simulink model "ES241A_MotAg2Meas"
settings: Solver=FixedStepDiscrete  SolverMode=SingleTasking  StartTime=0.0  StopTime=1  FixedStep=0.002  RelTol=1e-3
values from neighbouring files (symbols this model uses):
  ARCHGLBPRM_2PI_ULS_F32 = DataDict.Constant    [ES241A_MotAg2Meas_DataDict.m]
  FLTINJ_MOTAG2MEAS_MOTAG2MECL = DataDict.Constant    [ES241A_MotAg2Meas_DataDict.m]
  MOTAG2ANSINCOSFLTFAILSTEP_CNT_U16 = DataDict.Constant    [ES241A_MotAg2Meas_DataDict.m]
  MOTAG2ANSINCOSFLTPASSSTEP_CNT_U16 = DataDict.Constant    [ES241A_MotAg2Meas_DataDict.m]
  MotAg2MeasOffs = DataDict.Calibration    [ES241A_MotAg2Meas_DataDict.m]
  MOTAG2MECLMAX_MOTREV_F32 = DataDict.Constant    [ES241A_MotAg2Meas_DataDict.m]
  MOTAG2MECLMIN_MOTREV_F32 = DataDict.Constant    [ES241A_MotAg2Meas_DataDict.m]
  VALMAXERR_VOLTSQD_F32 = DataDict.Constant    [ES241A_MotAg2Meas_DataDict.m]
  VALMINERR_VOLTSQD_F32 = DataDict.Constant    [ES241A_MotAg2Meas_DataDict.m]
undefined symbols (not defined in the file or in its folder): NtcNr1, NtcSts1, sigbuilder_block
libraries: simulink x12, NxtrLim x2, FloatToFixd x1, NxtrMath x1
(part 2 of 3)

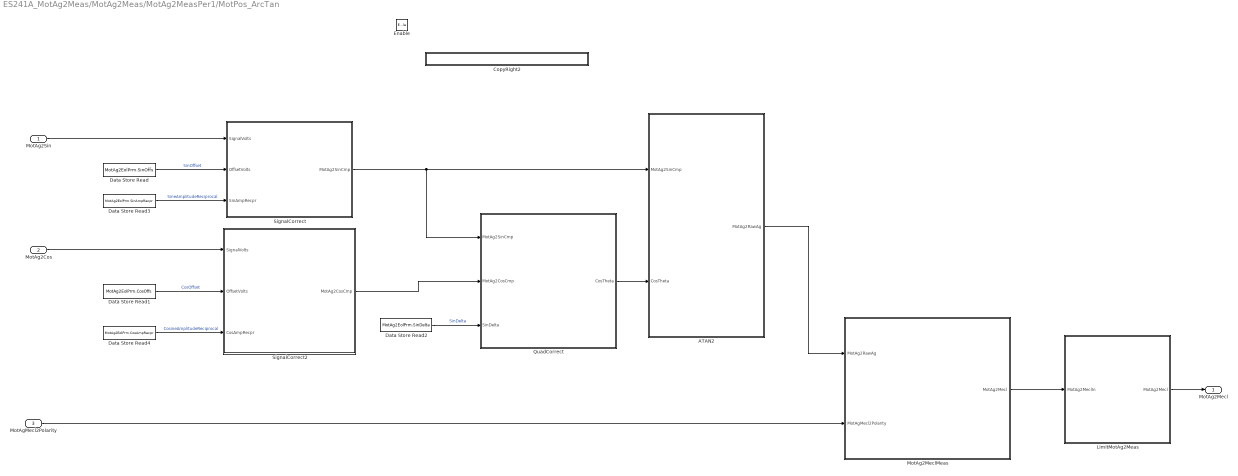
== system ES241A_MotAg2Meas/MotAg2Meas/MotAg2MeasPer1/MotPos_ArcTan ==
  MotAg2Sin : Inport
  MotAg2Cos : Inport  Port=2
  MotAgMecl2Polarity : Inport  RequirementInfo={} %GIDa_f88c60fe_1722_4e27_ab61_8a7da6a73543  Port=3
  Enable : EnablePort
  ATAN2 : Subsystem  RequirementInfo={'linktype_rmi_doors' '0000cf65 (/E-STEER Core/SubSystem Specifications/Electrical Actuator/Control Module/FDD Module Requirements/EA4/ES241A_MotAg2Meas)' '#ES241A_123' 'true' 'REQ: ES241A_123' '' } %GIDa_4a37e0cf_c570_47cf_a8a6_a1060e3c63ea  TreatAsAtomicUnit=on
  CopyRight2 : Subsystem  Description=|  mask(Copyright Information){none=on}
      | Copyright info block.                                               
      |                                                                     
      | Place copyright information at the top of every subsystem in design.
      mask prompts: none "No parameters"
      mask help: Place copyright information at the top of every subsystem in design.
      mask Display:
      | NxtrConf = 'Nexteer Confidential';
      | 
      | sys = bdroot; %handle for the current model ("system")
      | first = get_param(sys,'Created');
      | if(isempty(first))
      |     first = datestr(now,'yyyy');
      | else
      |     first = first(end-3:end);  %year is last four digits
      | end
      | 
      | last = get_param(sys,'LastModifiedDate');
      | if isempty(last)
      |     last = datestr(now,'yyyy');
      | else
      |     last = last(end-3:end);
      | end
      | 
      | if strcmp(first,last)
      |     fprintf('%s -- Copyright %s Nexteer',NxtrConf,first)
      | else
      |     fprintf('%s -- %s%s- %s Nexteer',NxtrConf,char(169),first,last)
      | end
  Data Store Read : DataStoreRead  DataStoreName=MotAg2EolPrm  DataStoreElements=MotAg2EolPrm.SinOffs
  Data Store Read1 : DataStoreRead  DataStoreName=MotAg2EolPrm  DataStoreElements=MotAg2EolPrm.CosOffs
  Data Store Read2 : DataStoreRead  DataStoreName=MotAg2EolPrm  DataStoreElements=MotAg2EolPrm.SinDelta
  Data Store Read3 : DataStoreRead  DataStoreName=MotAg2EolPrm  DataStoreElements=MotAg2EolPrm.SinAmpRecpr
  Data Store Read4 : DataStoreRead  DataStoreName=MotAg2EolPrm  DataStoreElements=MotAg2EolPrm.CosAmpRecpr
  LimitMotAg2Meas : Subsystem
  MotAg2MeclMeas : Subsystem  RequirementInfo="{}  %GIDa_155eb0a8_c2ed_490a_af1d_f8f4e19f97e7"  TreatAsAtomicUnit=on
  QuadCorrect : Subsystem  RequirementInfo={'linktype_rmi_doors' '0000cf65 (/E-STEER Core/SubSystem Specifications/Electrical Actuator/Control Module/FDD Module Requirements/EA4/ES241A_MotAg2Meas)' '#ES241A_121' 'true' 'REQ: ES241A_121' '' } %GIDa_3d78f2b2_5c94_409f_934c_8aefaaebd76d  TreatAsAtomicUnit=on
  SignalCorrect : Subsystem  RequirementInfo={'linktype_rmi_doors' '0000cf65 (/E-STEER Core/SubSystem Specifications/Electrical Actuator/Control Module/FDD Module Requirements/EA4/ES241A_MotAg2Meas)' '#ES241A_117' 'true' 'REQ: ES241A_117' '' } %GIDa_8d0c5619_ebe6_40e3_89d6_85a8ef0fbaf9
  SignalCorrect2 : Subsystem  RequirementInfo={'linktype_rmi_doors' '0000cf65 (/E-STEER Core/SubSystem Specifications/Electrical Actuator/Control Module/FDD Module Requirements/EA4/ES241A_MotAg2Meas)' '#ES241A_83' 'true' 'REQ: ES241A_83' '' } %GIDa_07f3fc20_adc4_4d19_a2a9_4772ed53a785
  MotAg2Mecl : Outport  RequirementInfo="{}  %GIDa_dd9bd2af_a5c1_4575_89a6_d173bd83c2f9"
  wires:
  SignalCorrect/1(MotAg2SinCmp) -> QuadCorrect/1(MotAg2SinCmp), ATAN2/1(MotAg2SinCmp)
  ATAN2/1(MotAg2RawAg) -> MotAg2MeclMeas/1(MotAg2RawAg)
  MotAg2Cos/1 -> SignalCorrect2/1(SignalVolts)
  MotAgMecl2Polarity/1 -> MotAg2MeclMeas/2(MotAgMecl2Polarity)
  SignalCorrect2/1(MotAg2CosCmp) -> QuadCorrect/2(MotAg2CosCmp)
  Data Store Read/1 -> SignalCorrect/2(OffsetVolts)  "SinOffset"
  Data Store Read3/1 -> SignalCorrect/3(SinAmpRecpr)  "SineAmplitudeReciprocal"
  Data Store Read1/1 -> SignalCorrect2/2(OffsetVolts)  "CosOffset"
  Data Store Read4/1 -> SignalCorrect2/3(CosAmpRecpr)  "CosineAmplitudeReciprocal"
  Data Store Read2/1 -> QuadCorrect/3(SinDelta)  "SinDelta"
  MotAg2Sin/1 -> SignalCorrect/1(SignalVolts)
  MotAg2MeclMeas/1(MotAg2Mecl) -> LimitMotAg2Meas/1(MotAg2MeclIn)
  LimitMotAg2Meas/1(MotAg2Mecl) -> MotAg2Mecl/1
  QuadCorrect/1(CosTheta) -> ATAN2/2(CosTheta)

== system ES241A_MotAg2Meas/MotAg2Meas/MotAg2MeasInit1/MotAg2EolPrm_GetErrorStatus/CopyRight2 ==

== system ES241A_MotAg2Meas/MotAg2Meas/MotAg2MeasInit1/NVM_NOK/CopyRight2 ==

== system ES241A_MotAg2Meas/MotAg2Meas/MotAg2MeasInit1/NVM_Ok/CopyRight2 ==

== system ES241A_MotAg2Meas/MotAg2Meas/MotAg2MeasPer1/AnalogMsbDiagnostics/CopyRight2 ==

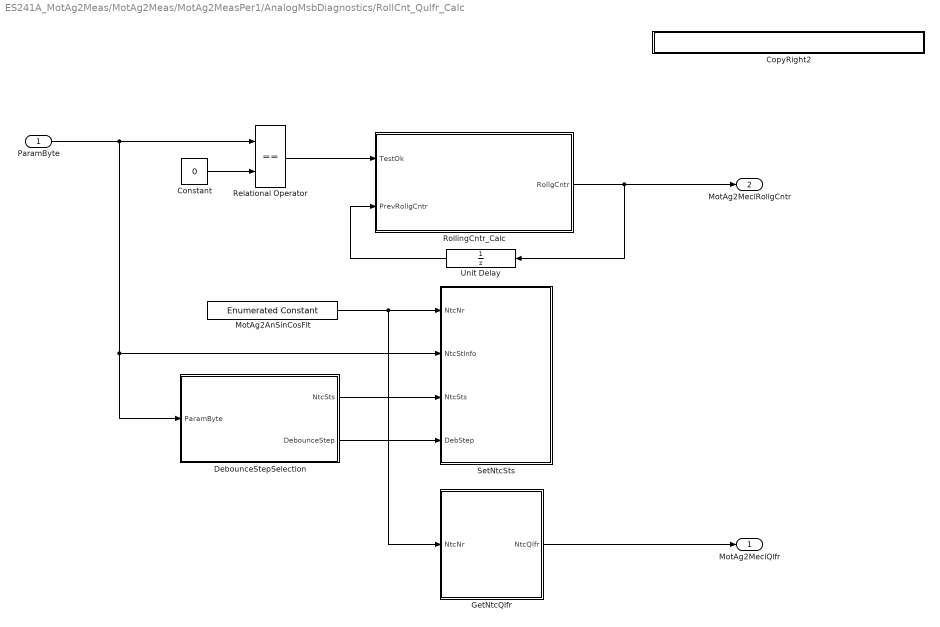
== system ES241A_MotAg2Meas/MotAg2Meas/MotAg2MeasPer1/AnalogMsbDiagnostics/RollCnt_Qulfr_Calc ==
  ParamByte : Inport
  Constant : Constant  Value=0
  CopyRight2 : Subsystem  Description=|  mask(Copyright Information){none=on}
      | Copyright info block.                                               
      |                                                                     
      | Place copyright information at the top of every subsystem in design.
      mask prompts: none "No parameters"
      mask help: Place copyright information at the top of every subsystem in design.
      mask Display:
      | NxtrConf = 'Nexteer Confidential';
      | 
      | sys = bdroot; %handle for the current model ("system")
      | first = get_param(sys,'Created');
      | if(isempty(first))
      |     first = datestr(now,'yyyy');
      | else
      |     first = first(end-3:end);  %year is last four digits
      | end
      | 
      | last = get_param(sys,'LastModifiedDate');
      | if isempty(last)
      |     last = datestr(now,'yyyy');
      | else
      |     last = last(end-3:end);
      | end
      | 
      | if strcmp(first,last)
      |     fprintf('%s -- Copyright %s Nexteer',NxtrConf,first)
      | else
      |     fprintf('%s -- %s%s- %s Nexteer',NxtrConf,char(169),first,last)
      | end
  DebounceStepSelection : Subsystem
  GetNtcQlfr : Subsystem  RequirementInfo={'linktype_rmi_doors' '0000cf65 (/E-STEER Core/SubSystem Specifications/Electrical Actuator/Control Module/FDD Module Requirements/EA4/ES241A_MotAg2Meas)' '#ES241A_136' 'true' 'REQ: ES241A_136' '' } %GIDa_6b67fe78_f19c_4eda_b14f_32aa673a2169
  MotAg2AnSinCosFlt : simulink/Sources/Enumerated Constant  OutDataTypeStr=Enum: NtcNr1  Value=NtcNr1.NTCNR_0X087  SampleTime=inf
  Relational Operator : RelationalOperator  Operator===  OutDataTypeStr=boolean
  RollingCntr_Calc : Stateflow chart  TreatAsAtomicUnit=on
  SetNtcSts : Subsystem  RequirementInfo={} %GIDa_9fe419b1_aead_4464_8eaa_fcc4c094b192
  Unit Delay : UnitDelay  SampleTime=-1  StateName=MotAg2MeclRollgCntrPrev  StateMustResolveToSignalObject=on
      settings: AttributesFormatString=%<StateName>
  MotAg2MeclQlfr : Outport
  MotAg2MeclRollgCntr : Outport  Port=2
  wires:
  ParamByte/1 -> Relational Operator/1, DebounceStepSelection/1(ParamByte), SetNtcSts/2(NtcStInfo)
  RollingCntr_Calc/1(RollgCntr) -> MotAg2MeclRollgCntr/1, Unit Delay/1
  DebounceStepSelection/2(DebounceStep) -> SetNtcSts/4(DebStep)
  MotAg2AnSinCosFlt/1 -> GetNtcQlfr/1(NtcNr), SetNtcSts/1(NtcNr)
  GetNtcQlfr/1(NtcQlfr) -> MotAg2MeclQlfr/1
  DebounceStepSelection/1(NtcSts) -> SetNtcSts/3(NtcSts)
  Relational Operator/1 -> RollingCntr_Calc/1(TestOk)
  Constant/1 -> Relational Operator/2
  Unit Delay/1 -> RollingCntr_Calc/2(PrevRollgCntr)

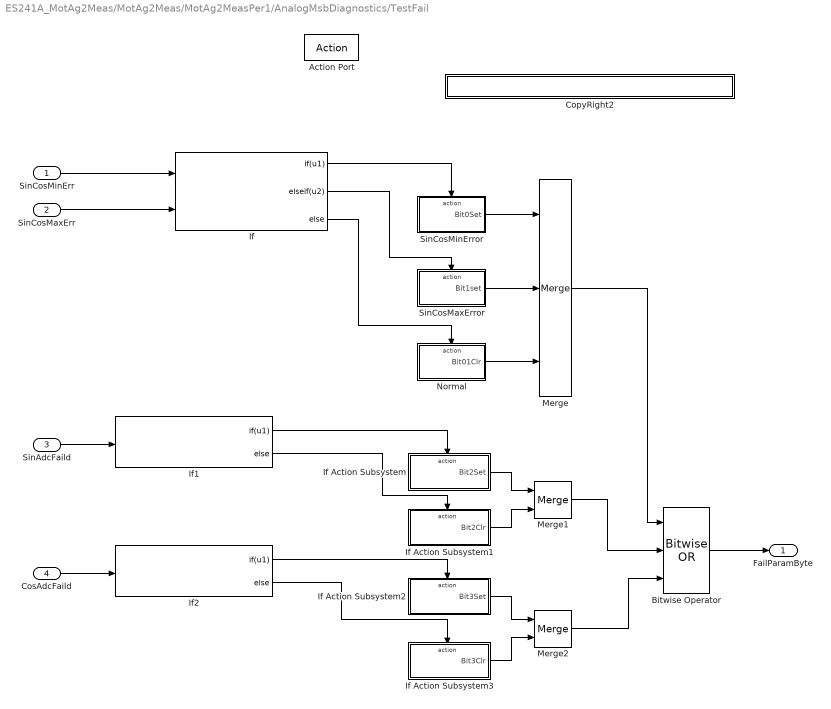
== system ES241A_MotAg2Meas/MotAg2Meas/MotAg2MeasPer1/AnalogMsbDiagnostics/TestFail ==
  SinCosMinErr : Inport
  SinCosMaxErr : Inport  Port=2
  SinAdcFaild : Inport  Port=3
  CosAdcFaild : Inport  Port=4
  Action Port : ActionPort  ActionType=then
  Bitwise Operator : simulink/Logic and Bit Operations/Bitwise Operator  logicop=OR  UseBitMask=off  NumInputPorts=3  BitMask=bin2dec('11011001')  BitMaskRealWorld=Stored Integer
  CopyRight2 : Subsystem  Description=|  mask(Copyright Information){none=on}
      | Copyright info block.                                               
      |                                                                     
      | Place copyright information at the top of every subsystem in design.
      mask prompts: none "No parameters"
      mask help: Place copyright information at the top of every subsystem in design.
      mask Display:
      | NxtrConf = 'Nexteer Confidential';
      | 
      | sys = bdroot; %handle for the current model ("system")
      | first = get_param(sys,'Created');
      | if(isempty(first))
      |     first = datestr(now,'yyyy');
      | else
      |     first = first(end-3:end);  %year is last four digits
      | end
      | 
      | last = get_param(sys,'LastModifiedDate');
      | if isempty(last)
      |     last = datestr(now,'yyyy');
      | else
      |     last = last(end-3:end);
      | end
      | 
      | if strcmp(first,last)
      |     fprintf('%s -- Copyright %s Nexteer',NxtrConf,first)
      | else
      |     fprintf('%s -- %s%s- %s Nexteer',NxtrConf,char(169),first,last)
      | end
  If : If  RequirementInfo={} %GIDa_a9e4a426_b13f_48ac_85a4_f1708270da02  NumInputs=2  IfExpression=u1  ElseIfExpressions=u2
  If Action Subsystem : Subsystem  RequirementInfo={'linktype_rmi_doors' '0000cf65 (/E-STEER Core/SubSystem Specifications/Electrical Actuator/Control Module/FDD Module Requirements/EA4/ES241A_MotAg2Meas)' '#ES241A_149' 'true' 'REQ: ES241A_149' '' } %GIDa_afb555f9_4864_4292_98a1_720bafda0c91  TreatAsAtomicUnit=on
  If Action Subsystem1 : Subsystem  RequirementInfo={'linktype_rmi_doors' '0000cf65 (/E-STEER Core/SubSystem Specifications/Electrical Actuator/Control Module/FDD Module Requirements/EA4/ES241A_MotAg2Meas)' '#ES241A_149' 'true' 'REQ: ES241A_149' '' } %GIDa_7a5d096e_f46e_4b81_973a_a988b07ea5da  TreatAsAtomicUnit=on
  If Action Subsystem2 : Subsystem  RequirementInfo={'linktype_rmi_doors' '0000cf65 (/E-STEER Core/SubSystem Specifications/Electrical Actuator/Control Module/FDD Module Requirements/EA4/ES241A_MotAg2Meas)' '#ES241A_150' 'true' 'REQ: ES241A_150' '' } %GIDa_1a2e8224_376f_4f7e_a8de_e2f9f89e8409  TreatAsAtomicUnit=on
  If Action Subsystem3 : Subsystem  RequirementInfo={'linktype_rmi_doors' '0000cf65 (/E-STEER Core/SubSystem Specifications/Electrical Actuator/Control Module/FDD Module Requirements/EA4/ES241A_MotAg2Meas)' '#ES241A_150' 'true' 'REQ: ES241A_150' '' } %GIDa_804518a5_ac45_4ee5_ad42_fdad3805a040  TreatAsAtomicUnit=on
  If1 : If  RequirementInfo={} %GIDa_4ac208ba_4fea_48e5_9089_44454d5bb31e  IfExpression=u1
  If2 : If  RequirementInfo={} %GIDa_95f3580d_6d83_47db_9291_d4b911f8f78c  IfExpression=u1
  Merge : Merge  Inputs=3
  Merge1 : Merge
  Merge2 : Merge
  Normal : Subsystem  RequirementInfo={'linktype_rmi_doors' '0000cf65 (/E-STEER Core/SubSystem Specifications/Electrical Actuator/Control Module/FDD Module Requirements/EA4/ES241A_MotAg2Meas)' '#ES241A_132' 'true' 'REQ: ES241A_132' '' ; 'linktype_rmi_doors' '0000cf65 (/E-STEER Core/SubSystem Specifications/Electrical Actuator/Control Module/FDD Module Requirements/EA4/ES241A_MotAg2Meas)' '#ES241A_133' 'true' 'REQ: ES241A_133' '' } %GIDa_7888af4c_2405_41f3_8422_50cb1e840d88  TreatAsAtomicUnit=on
  SinCosMaxError : Subsystem  RequirementInfo={'linktype_rmi_doors' '0000cf65 (/E-STEER Core/SubSystem Specifications/Electrical Actuator/Control Module/FDD Module Requirements/EA4/ES241A_MotAg2Meas)' '#ES241A_132' 'true' 'REQ: ES241A_132' '' } %GIDa_2a13378d_a5ac_4539_9cf9_334d2a433c6e  TreatAsAtomicUnit=on
  SinCosMinError : Subsystem  RequirementInfo={'linktype_rmi_doors' '0000cf65 (/E-STEER Core/SubSystem Specifications/Electrical Actuator/Control Module/FDD Module Requirements/EA4/ES241A_MotAg2Meas)' '#ES241A_133' 'true' 'REQ: ES241A_133' '' } %GIDa_e3821827_fad7_4466_9101_6350f28db25f  TreatAsAtomicUnit=on
  FailParamByte : Outport
  wires:
  SinCosMinErr/1 -> If/1
  If/1 -> SinCosMinError/Action
  SinCosMinError/1(Bit0Set) -> Merge/1
  SinCosMaxError/1(Bit1set) -> Merge/2
  SinCosMaxErr/1 -> If/2
  If/2 -> SinCosMaxError/Action
  SinAdcFaild/1 -> If1/1
  CosAdcFaild/1 -> If2/1
  If/3 -> Normal/Action
  Normal/1(Bit01Clr) -> Merge/3
  If1/1 -> If Action Subsystem/Action
  If1/2 -> If Action Subsystem1/Action
  If2/1 -> If Action Subsystem2/Action
  If2/2 -> If Action Subsystem3/Action
  If Action Subsystem/1(Bit2Set) -> Merge1/1
  If Action Subsystem1/1(Bit2Clr) -> Merge1/2
  If Action Subsystem2/1(Bit3Set) -> Merge2/1
  If Action Subsystem3/1(Bit3Clr) -> Merge2/2
  Merge1/1 -> Bitwise Operator/2
  Merge2/1 -> Bitwise Operator/3
  Bitwise Operator/1 -> FailParamByte/1
  Merge/1 -> Bitwise Operator/1

== system ES241A_MotAg2Meas/MotAg2Meas/MotAg2MeasPer1/AnalogMsbDiagnostics/TestPass ==
  Action Port : ActionPort  ActionType=else
  Constant : Constant  Value=0  OutDataTypeStr=uint8
      settings: AttributesFormatString=%<OutDataTypeStr>
  CopyRight2 : Subsystem  Description=|  mask(Copyright Information){none=on}
      | Copyright info block.                                               
      |                                                                     
      | Place copyright information at the top of every subsystem in design.
      mask prompts: none "No parameters"
      mask help: Place copyright information at the top of every subsystem in design.
      mask Display:
      | NxtrConf = 'Nexteer Confidential';
      | 
      | sys = bdroot; %handle for the current model ("system")
      | first = get_param(sys,'Created');
      | if(isempty(first))
      |     first = datestr(now,'yyyy');
      | else
      |     first = first(end-3:end);  %year is last four digits
      | end
      | 
      | last = get_param(sys,'LastModifiedDate');
      | if isempty(last)
      |     last = datestr(now,'yyyy');
      | else
      |     last = last(end-3:end);
      | end
      | 
      | if strcmp(first,last)
      |     fprintf('%s -- Copyright %s Nexteer',NxtrConf,first)
      | else
      |     fprintf('%s -- %s%s- %s Nexteer',NxtrConf,char(169),first,last)
      | end
  PassParamByte : Outport
  wires:
  Constant/1 -> PassParamByte/1  "ParamByte"

== system ES241A_MotAg2Meas/MotAg2Meas/MotAg2MeasPer1/FltInj_f32/CopyRight2 ==

== system ES241A_MotAg2Meas/MotAg2Meas/MotAg2MeasPer1/MotAngleMechRevJdgmnt/CopyRight2 ==

== system ES241A_MotAg2Meas/MotAg2Meas/MotAg2MeasPer1/MotAngleMechRevJdgmnt/TesOk_Fail ==
  In1 : Inport
  Action Port : ActionPort  ActionType=else
  CopyRight2 : Subsystem  Description=|  mask(Copyright Information){none=on}
      | Copyright info block.                                               
      |                                                                     
      | Place copyright information at the top of every subsystem in design.
      mask prompts: none "No parameters"
      mask help: Place copyright information at the top of every subsystem in design.
      mask Display:
      | NxtrConf = 'Nexteer Confidential';
      | 
      | sys = bdroot; %handle for the current model ("system")
      | first = get_param(sys,'Created');
      | if(isempty(first))
      |     first = datestr(now,'yyyy');
      | else
      |     first = first(end-3:end);  %year is last four digits
      | end
      | 
      | last = get_param(sys,'LastModifiedDate');
      | if isempty(last)
      |     last = datestr(now,'yyyy');
      | else
      |     last = last(end-3:end);
      | end
      | 
      | if strcmp(first,last)
      |     fprintf('%s -- Copyright %s Nexteer',NxtrConf,first)
      | else
      |     fprintf('%s -- %s%s- %s Nexteer',NxtrConf,char(169),first,last)
      | end
  Out1 : Outport
  wires:
  In1/1 -> Out1/1

== system ES241A_MotAg2Meas/MotAg2Meas/MotAg2MeasPer1/MotAngleMechRevJdgmnt/TesOk_Pass ==
  In1 : Inport
  Action Port : ActionPort  ActionType=then
  CopyRight2 : Subsystem  Description=|  mask(Copyright Information){none=on}
      | Copyright info block.                                               
      |                                                                     
      | Place copyright information at the top of every subsystem in design.
      mask prompts: none "No parameters"
      mask help: Place copyright information at the top of every subsystem in design.
      mask Display:
      | NxtrConf = 'Nexteer Confidential';
      | 
      | sys = bdroot; %handle for the current model ("system")
      | first = get_param(sys,'Created');
      | if(isempty(first))
      |     first = datestr(now,'yyyy');
      | else
      |     first = first(end-3:end);  %year is last four digits
      | end
      | 
      | last = get_param(sys,'LastModifiedDate');
      | if isempty(last)
      |     last = datestr(now,'yyyy');
      | else
      |     last = last(end-3:end);
      | end
      | 
      | if strcmp(first,last)
      |     fprintf('%s -- Copyright %s Nexteer',NxtrConf,first)
      | else
      |     fprintf('%s -- %s%s- %s Nexteer',NxtrConf,char(169),first,last)
      | end
  Out1 : Outport
  wires:
  In1/1 -> Out1/1

== system ES241A_MotAg2Meas/MotAg2Meas/MotAg2MeasPer1/MotPos_ArcTan/ATAN2 ==
  note: The motor angle mechanical output is 0 to 1 motor mechancial revolutions.
      |  Zero represents the point where sine is 0 and cosine is 1
  MotAg2SinCmp : Inport
  CosTheta : Inport  Port=2
  Arctan2_f32 : NxtrMath/Arctan2_f32  SFunctionSpec=single y1 = Arctan2_f32(single u1, single u2)
      settings: AttributesFormatString=%<MaskType>
  Constant5 : Constant  Value=ARCHGLBPRM_2PI_ULS_F32
  CopyRight2 : Subsystem  Description=|  mask(Copyright Information){none=on}
      | Copyright info block.                                               
      |                                                                     
      | Place copyright information at the top of every subsystem in design.
      mask prompts: none "No parameters"
      mask help: Place copyright information at the top of every subsystem in design.
      mask Display:
      | NxtrConf = 'Nexteer Confidential';
      | 
      | sys = bdroot; %handle for the current model ("system")
      | first = get_param(sys,'Created');
      | if(isempty(first))
      |     first = datestr(now,'yyyy');
      | else
      |     first = first(end-3:end);  %year is last four digits
      | end
      | 
      | last = get_param(sys,'LastModifiedDate');
      | if isempty(last)
      |     last = datestr(now,'yyyy');
      | else
      |     last = last(end-3:end);
      | end
      | 
      | if strcmp(first,last)
      |     fprintf('%s -- Copyright %s Nexteer',NxtrConf,first)
      | else
      |     fprintf('%s -- %s%s- %s Nexteer',NxtrConf,char(169),first,last)
      | end
  Divide2 : Product  Inputs=*/
  MotAg2RawAg : Outport
  wires:
  Constant5/1 -> Divide2/2
  CosTheta/1 -> Arctan2_f32/2
  MotAg2SinCmp/1 -> Arctan2_f32/1
  Divide2/1 -> MotAg2RawAg/1
  Arctan2_f32/1 -> Divide2/1

== system ES241A_MotAg2Meas/MotAg2Meas/MotAg2MeasPer1/MotPos_ArcTan/CopyRight2 ==

== system ES241A_MotAg2Meas/MotAg2Meas/MotAg2MeasPer1/MotPos_ArcTan/LimitMotAg2Meas ==
  MotAg2MeclIn : Inport
  CopyRight2 : Subsystem  Description=|  mask(Copyright Information){none=on}
      | Copyright info block.                                               
      |                                                                     
      | Place copyright information at the top of every subsystem in design.
      mask prompts: none "No parameters"
      mask help: Place copyright information at the top of every subsystem in design.
      mask Display:
      | NxtrConf = 'Nexteer Confidential';
      | 
      | sys = bdroot; %handle for the current model ("system")
      | first = get_param(sys,'Created');
      | if(isempty(first))
      |     first = datestr(now,'yyyy');
      | else
      |     first = first(end-3:end);  %year is last four digits
      | end
      | 
      | last = get_param(sys,'LastModifiedDate');
      | if isempty(last)
      |     last = datestr(now,'yyyy');
      | else
      |     last = last(end-3:end);
      | end
      | 
      | if strcmp(first,last)
      |     fprintf('%s -- Copyright %s Nexteer',NxtrConf,first)
      | else
      |     fprintf('%s -- %s%s- %s Nexteer',NxtrConf,char(169),first,last)
      | end
  NormalizeMotAg2Mecl : Stateflow chart  TreatAsAtomicUnit=on
  MotAg2Mecl : Outport
  wires:
  NormalizeMotAg2Mecl/1(MotAg2Mecl) -> MotAg2Mecl/1
  MotAg2MeclIn/1 -> NormalizeMotAg2Mecl/1(MotAg2MeclIn)

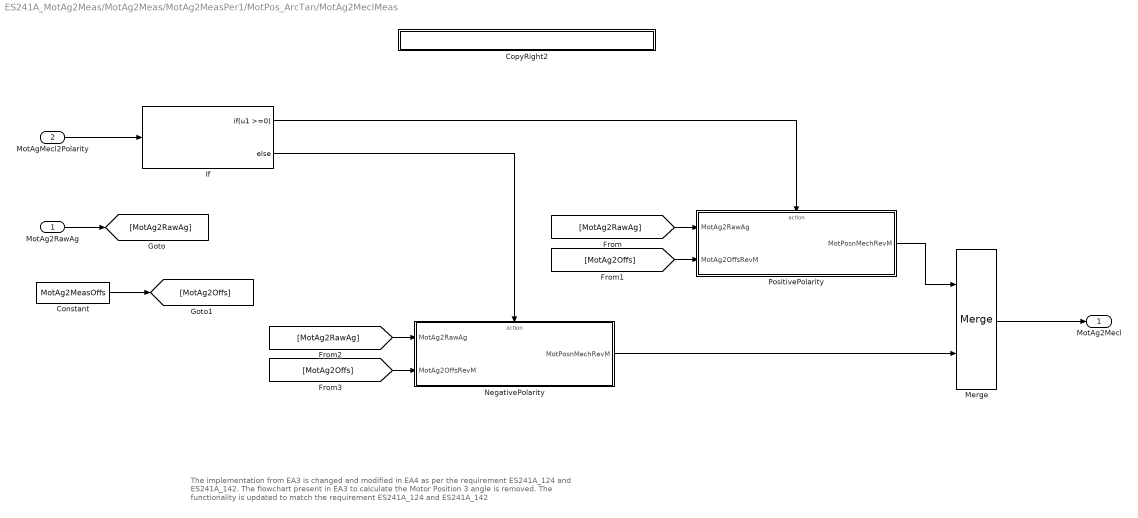
== system ES241A_MotAg2Meas/MotAg2Meas/MotAg2MeasPer1/MotPos_ArcTan/MotAg2MeclMeas ==
  note: The implementation from EA3 is changed and modified in EA4 as per the requirement ES241A_124 and ES241A_142. The flowchart present in EA3 to calculate the
      | Motor Position 3 angle is removed. The functionality is updated to match the requirement  ES241A_124 and ES241A_142
  MotAg2RawAg : Inport
  MotAgMecl2Polarity : Inport  RequirementInfo={} %GIDa_48baabf2_6d88_4062_b7d2_0aa56f82b9bc  Port=2
  Constant : Constant  Value=MotAg2MeasOffs
  CopyRight2 : Subsystem  Description=|  mask(Copyright Information){none=on}
      | Copyright info block.                                               
      |                                                                     
      | Place copyright information at the top of every subsystem in design.
      mask prompts: none "No parameters"
      mask help: Place copyright information at the top of every subsystem in design.
      mask Display:
      | NxtrConf = 'Nexteer Confidential';
      | 
      | sys = bdroot; %handle for the current model ("system")
      | first = get_param(sys,'Created');
      | if(isempty(first))
      |     first = datestr(now,'yyyy');
      | else
      |     first = first(end-3:end);  %year is last four digits
      | end
      | 
      | last = get_param(sys,'LastModifiedDate');
      | if isempty(last)
      |     last = datestr(now,'yyyy');
      | else
      |     last = last(end-3:end);
      | end
      | 
      | if strcmp(first,last)
      |     fprintf('%s -- Copyright %s Nexteer',NxtrConf,first)
      | else
      |     fprintf('%s -- %s%s- %s Nexteer',NxtrConf,char(169),first,last)
      | end
  If : If  IfExpression=u1 >=0
  Merge : Merge
  NegativePolarity : Subsystem  RequirementInfo={'linktype_rmi_doors' '0000cf65 (/E-STEER Core/SubSystem Specifications/Electrical Actuator/Control Module/FDD Module Requirements/EA4/ES241A_MotAg2Meas)' '#ES241A_142' 'true' 'REQ: ES241A_142' '' } %GIDa_a914b3a1_42a7_4120_8075_f930cacf512b  TreatAsAtomicUnit=on
  PositivePolarity : Subsystem  RequirementInfo={'linktype_rmi_doors' '0000cf65 (/E-STEER Core/SubSystem Specifications/Electrical Actuator/Control Module/FDD Module Requirements/EA4/ES241A_MotAg2Meas)' '#ES241A_124' 'true' 'REQ: ES241A_124' '' } %GIDa_14d2658d_6583_4367_a092_906faf885405  TreatAsAtomicUnit=on
  MotAg2Mecl : Outport
  wires:
  MotAgMecl2Polarity/1 -> If/1
  If/1 -> PositivePolarity/Action
  MotAg2RawAg/1 -> [MotAg2RawAg]
  Constant/1 -> [MotAg2Offs]
  [MotAg2RawAg] -> PositivePolarity/1(MotAg2RawAg)
  [MotAg2Offs] -> PositivePolarity/2(MotAg2OffsRevM)
  [MotAg2Offs] -> NegativePolarity/2(MotAg2OffsRevM)
  [MotAg2RawAg] -> NegativePolarity/1(MotAg2RawAg)
  If/2 -> NegativePolarity/Action
  NegativePolarity/1(MotPosnMechRevM) -> Merge/2
  PositivePolarity/1(MotPosnMechRevM) -> Merge/1
  Merge/1 -> MotAg2Mecl/1

== system ES241A_MotAg2Meas/MotAg2Meas/MotAg2MeasPer1/MotPos_ArcTan/QuadCorrect ==
  MotAg2SinCmp : Inport
  MotAg2CosCmp : Inport  Port=2
  SinDelta : Inport  Port=3
  Add : Sum
  CopyRight2 : Subsystem  Description=|  mask(Copyright Information){none=on}
      | Copyright info block.                                               
      |                                                                     
      | Place copyright information at the top of every subsystem in design.
      mask prompts: none "No parameters"
      mask help: Place copyright information at the top of every subsystem in design.
      mask Display:
      | NxtrConf = 'Nexteer Confidential';
      | 
      | sys = bdroot; %handle for the current model ("system")
      | first = get_param(sys,'Created');
      | if(isempty(first))
      |     first = datestr(now,'yyyy');
      | else
      |     first = first(end-3:end);  %year is last four digits
      | end
      | 
      | last = get_param(sys,'LastModifiedDate');
      | if isempty(last)
      |     last = datestr(now,'yyyy');
      | else
      |     last = last(end-3:end);
      | end
      | 
      | if strcmp(first,last)
      |     fprintf('%s -- Copyright %s Nexteer',NxtrConf,first)
      | else
      |     fprintf('%s -- %s%s- %s Nexteer',NxtrConf,char(169),first,last)
      | end
  Product : Product
  CosTheta : Outport
  wires:
  Add/1 -> CosTheta/1
  MotAg2CosCmp/1 -> Add/2
  Product/1 -> Add/1
  SinDelta/1 -> Product/2
  MotAg2SinCmp/1 -> Product/1

== system ES241A_MotAg2Meas/MotAg2Meas/MotAg2MeasPer1/MotPos_ArcTan/SignalCorrect ==
  SignalVolts : Inport  RequirementInfo={} %GIDa_4d46c49c_d29f_4dc1_b59e_11e8df28708d
  OffsetVolts : Inport  RequirementInfo={} %GIDa_9e934ba0_a188_47b4_99f1_79ba1a75ce9a  Port=2
  SinAmpRecpr : Inport  RequirementInfo={} %GIDa_8d1ecce4_4bc9_4bb4_840a_e49fc33b0ef5  Port=3
  CopyRight2 : Subsystem  Description=|  mask(Copyright Information){none=on}
      | Copyright info block.                                               
      |                                                                     
      | Place copyright information at the top of every subsystem in design.
      mask prompts: none "No parameters"
      mask help: Place copyright information at the top of every subsystem in design.
      mask Display:
      | NxtrConf = 'Nexteer Confidential';
      | 
      | sys = bdroot; %handle for the current model ("system")
      | first = get_param(sys,'Created');
      | if(isempty(first))
      |     first = datestr(now,'yyyy');
      | else
      |     first = first(end-3:end);  %year is last four digits
      | end
      | 
      | last = get_param(sys,'LastModifiedDate');
      | if isempty(last)
      |     last = datestr(now,'yyyy');
      | else
      |     last = last(end-3:end);
      | end
      | 
      | if strcmp(first,last)
      |     fprintf('%s -- Copyright %s Nexteer',NxtrConf,first)
      | else
      |     fprintf('%s -- %s%s- %s Nexteer',NxtrConf,char(169),first,last)
      | end
  Product : Product  RequirementInfo={} %GIDa_0ef12946_9e43_4e3e_9be5_386efad71f39
  Subtract : Sum  RequirementInfo={} %GIDa_4416986d_03ec_4524_9b9b_74a0c5b5f571  Inputs=+-
  MotAg2SinCmp : Outport
  wires:
  SignalVolts/1 -> Subtract/1
  Product/1 -> MotAg2SinCmp/1
  OffsetVolts/1 -> Subtract/2
  Subtract/1 -> Product/1
  SinAmpRecpr/1 -> Product/2

== system ES241A_MotAg2Meas/MotAg2Meas/MotAg2MeasPer1/MotPos_ArcTan/SignalCorrect2 ==
  SignalVolts : Inport  RequirementInfo={} %GIDa_74c68c6c_83f0_4816_b347_ac892d192fe3
  OffsetVolts : Inport  RequirementInfo={} %GIDa_4b7d013a_d637_41e8_87d4_3148678fec06  Port=2
  CosAmpRecpr : Inport  RequirementInfo={} %GIDa_71036c75_e094_47dd_88f8_0fa03d2893af  Port=3
  CopyRight2 : Subsystem  Description=|  mask(Copyright Information){none=on}
      | Copyright info block.                                               
      |                                                                     
      | Place copyright information at the top of every subsystem in design.
      mask prompts: none "No parameters"
      mask help: Place copyright information at the top of every subsystem in design.
      mask Display:
      | NxtrConf = 'Nexteer Confidential';
      | 
      | sys = bdroot; %handle for the current model ("system")
      | first = get_param(sys,'Created');
      | if(isempty(first))
      |     first = datestr(now,'yyyy');
      | else
      |     first = first(end-3:end);  %year is last four digits
      | end
      | 
      | last = get_param(sys,'LastModifiedDate');
      | if isempty(last)
      |     last = datestr(now,'yyyy');
      | else
      |     last = last(end-3:end);
      | end
      | 
      | if strcmp(first,last)
      |     fprintf('%s -- Copyright %s Nexteer',NxtrConf,first)
      | else
      |     fprintf('%s -- %s%s- %s Nexteer',NxtrConf,char(169),first,last)
      | end
  Product1 : Product  RequirementInfo={} %GIDa_99c3bc93_10b5_4d9d_b5c6_b1c10ee09e28
  Subtract1 : Sum  RequirementInfo={} %GIDa_dc70e87b_cdd9_4af6_b253_20d9dc932e67  Inputs=+-  OutDataTypeStr=Inherit: Inherit via back propagation
  MotAg2CosCmp : Outport
  wires:
  Product1/1 -> MotAg2CosCmp/1
  SignalVolts/1 -> Subtract1/1
  OffsetVolts/1 -> Subtract1/2
  Subtract1/1 -> Product1/1
  CosAmpRecpr/1 -> Product1/2

== system ES241A_MotAg2Meas/MotAg2Meas/MotAg2MeasPer1/AnalogMsbDiagnostics/RollCnt_Qulfr_Calc/CopyRight2 ==

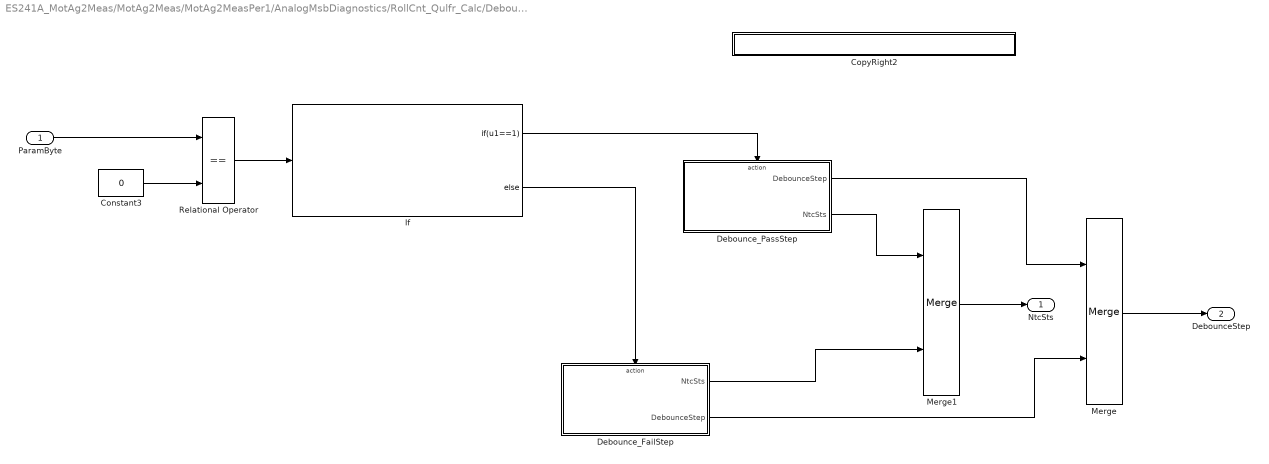
== system ES241A_MotAg2Meas/MotAg2Meas/MotAg2MeasPer1/AnalogMsbDiagnostics/RollCnt_Qulfr_Calc/DebounceStepSelection ==
  ParamByte : Inport
  Constant3 : Constant  Value=0
  CopyRight2 : Subsystem  Description=|  mask(Copyright Information){none=on}
      | Copyright info block.                                               
      |                                                                     
      | Place copyright information at the top of every subsystem in design.
      mask prompts: none "No parameters"
      mask help: Place copyright information at the top of every subsystem in design.
      mask Display:
      | NxtrConf = 'Nexteer Confidential';
      | 
      | sys = bdroot; %handle for the current model ("system")
      | first = get_param(sys,'Created');
      | if(isempty(first))
      |     first = datestr(now,'yyyy');
      | else
      |     first = first(end-3:end);  %year is last four digits
      | end
      | 
      | last = get_param(sys,'LastModifiedDate');
      | if isempty(last)
      |     last = datestr(now,'yyyy');
      | else
      |     last = last(end-3:end);
      | end
      | 
      | if strcmp(first,last)
      |     fprintf('%s -- Copyright %s Nexteer',NxtrConf,first)
      | else
      |     fprintf('%s -- %s%s- %s Nexteer',NxtrConf,char(169),first,last)
      | end
  Debounce_FailStep : Subsystem  TreatAsAtomicUnit=on
  Debounce_PassStep : Subsystem  TreatAsAtomicUnit=on
  If : If  IfExpression=u1==1
  Merge : Merge
  Merge1 : Merge
  Relational Operator : RelationalOperator  Operator===  OutDataTypeStr=boolean
  NtcSts : Outport
  DebounceStep : Outport  Port=2
  wires:
  If/1 -> Debounce_PassStep/Action
  If/2 -> Debounce_FailStep/Action
  Debounce_PassStep/1(DebounceStep) -> Merge/1
  Debounce_FailStep/2(DebounceStep) -> Merge/2
  Merge/1 -> DebounceStep/1
  Constant3/1 -> Relational Operator/2
  ParamByte/1 -> Relational Operator/1
  Relational Operator/1 -> If/1
  Debounce_PassStep/2(NtcSts) -> Merge1/1
  Debounce_FailStep/1(NtcSts) -> Merge1/2
  Merge1/1 -> NtcSts/1

== system ES241A_MotAg2Meas/MotAg2Meas/MotAg2MeasPer1/AnalogMsbDiagnostics/RollCnt_Qulfr_Calc/GetNtcQlfr ==
  NtcNr : Inport
  CopyRight2 : Subsystem  Description=|  mask(Copyright Information){none=on}
      | Copyright info block.                                               
      |                                                                     
      | Place copyright information at the top of every subsystem in design.
      mask prompts: none "No parameters"
      mask help: Place copyright information at the top of every subsystem in design.
      mask Display:
      | NxtrConf = 'Nexteer Confidential';
      | 
      | sys = bdroot; %handle for the current model ("system")
      | first = get_param(sys,'Created');
      | first = first(end-3:end);  %year is last four digits
      | 
      | last = get_param(sys,'LastModifiedDate');
      | if isempty(last)
      |     last = datestr(now,'yyyy');
      | else
      |     last = last(end-3:end);
      | end
      | 
      | if strcmp(first,last)
      |     fprintf('%s -- Copyright %s Nexteer',NxtrConf,first)
      | else
      |     fprintf('%s -- %s%s- %s Nexteer',NxtrConf,char(169),first,last)
      | end
  Data Store Read : DataStoreRead  DataStoreName=Ntc0x087Qlfr
  Terminator : Terminator
  NtcQlfr : Outport
  wires:
  NtcNr/1 -> Terminator/1
  Data Store Read/1 -> NtcQlfr/1

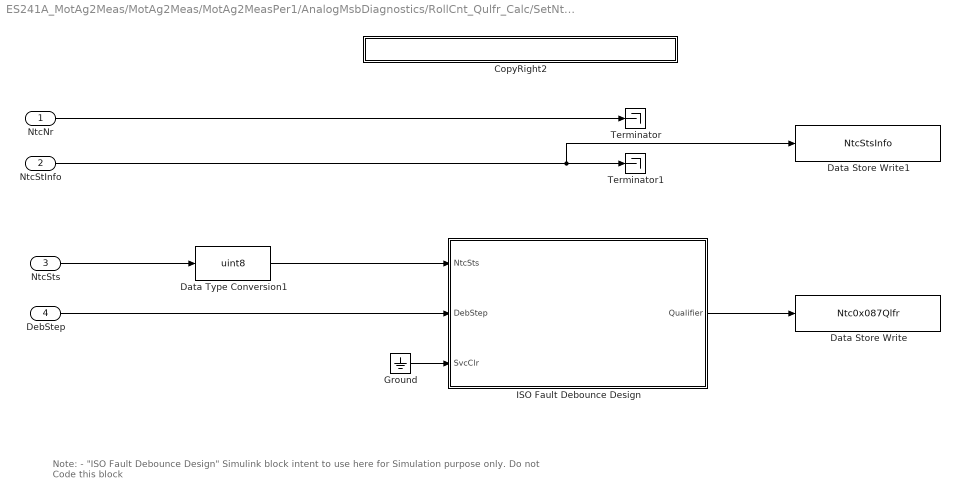
== system ES241A_MotAg2Meas/MotAg2Meas/MotAg2MeasPer1/AnalogMsbDiagnostics/RollCnt_Qulfr_Calc/SetNtcSts ==
  note: Note:
      |
      | - "ISO Fault Debounce Design" Simulink block intent to use here for Simulation purpose only. Do not Code this block
  NtcNr : Inport
  NtcStInfo : Inport  Port=2
  NtcSts : Inport  Port=3
  DebStep : Inport  Port=4
  CopyRight2 : Subsystem  Description=|  mask(Copyright Information){none=on}
      | Copyright info block.                                               
      |                                                                     
      | Place copyright information at the top of every subsystem in design.
      mask prompts: none "No parameters"
      mask help: Place copyright information at the top of every subsystem in design.
      mask Display:
      | NxtrConf = 'Nexteer Confidential';
      | 
      | sys = bdroot; %handle for the current model ("system")
      | first = get_param(sys,'Created');
      | first = first(end-3:end);  %year is last four digits
      | 
      | last = get_param(sys,'LastModifiedDate');
      | if isempty(last)
      |     last = datestr(now,'yyyy');
      | else
      |     last = last(end-3:end);
      | end
      | 
      | if strcmp(first,last)
      |     fprintf('%s -- Copyright %s Nexteer',NxtrConf,first)
      | else
      |     fprintf('%s -- %s%s- %s Nexteer',NxtrConf,char(169),first,last)
      | end
  Data Store Write : DataStoreWrite  DataStoreName=Ntc0x087Qlfr
  Data Store Write1 : DataStoreWrite  DataStoreName=NtcStsInfo
  Data Type Conversion1 : DataTypeConversion  OutDataTypeStr=uint8
  Ground : Ground
  ISO Fault Debounce Design : Stateflow chart  TreatAsAtomicUnit=on
      settings: AttributesFormatString=|
      | Simulation Purpose Only.
      | Do Not Code this block
      | Diagnostic Manager Owns this requirement
  Terminator : Terminator
  Terminator1 : Terminator
  wires:
  NtcNr/1 -> Terminator/1
  NtcSts/1 -> Data Type Conversion1/1
  DebStep/1 -> ISO Fault Debounce Design/2(DebStep)
  NtcStInfo/1 -> Data Store Write1/1, Terminator1/1
  Ground/1 -> ISO Fault Debounce Design/3(SvcClr)
  ISO Fault Debounce Design/1(Qualifier) -> Data Store Write/1
  Data Type Conversion1/1 -> ISO Fault Debounce Design/1(NtcSts)

== system ES241A_MotAg2Meas/MotAg2Meas/MotAg2MeasPer1/AnalogMsbDiagnostics/TestFail/CopyRight2 ==

== system ES241A_MotAg2Meas/MotAg2Meas/MotAg2MeasPer1/AnalogMsbDiagnostics/TestFail/If Action Subsystem ==
  Action Port : ActionPort  ActionType=then
  Bit Set : simulink/Logic and Bit Operations/Bit Set  iBit=2
  Constant1 : Constant  Value=0  OutDataTypeStr=uint8
      settings: AttributesFormatString=%<OutDataTypeStr>
  CopyRight2 : Subsystem  Description=|  mask(Copyright Information){none=on}
      | Copyright info block.                                               
      |                                                                     
      | Place copyright information at the top of every subsystem in design.
      mask prompts: none "No parameters"
      mask help: Place copyright information at the top of every subsystem in design.
      mask Display:
      | NxtrConf = 'Nexteer Confidential';
      | 
      | sys = bdroot; %handle for the current model ("system")
      | first = get_param(sys,'Created');
      | first = first(end-3:end);  %year is last four digits
      | 
      | last = get_param(sys,'LastModifiedDate');
      | if isempty(last)
      |     last = datestr(now,'yyyy');
      | else
      |     last = last(end-3:end);
      | end
      | 
      | if strcmp(first,last)
      |     fprintf('%s -- Copyright %s Nexteer',NxtrConf,first)
      | else
      |     fprintf('%s -- %s%s- %s Nexteer',NxtrConf,char(169),first,last)
      | end
  Bit2Set : Outport
  wires:
  Constant1/1 -> Bit Set/1
  Bit Set/1 -> Bit2Set/1

== system ES241A_MotAg2Meas/MotAg2Meas/MotAg2MeasPer1/AnalogMsbDiagnostics/TestFail/If Action Subsystem1 ==
  Action Port : ActionPort  ActionType=else
  Constant1 : Constant  Value=0  OutDataTypeStr=uint8
      settings: AttributesFormatString=%<OutDataTypeStr>
  CopyRight2 : Subsystem  Description=|  mask(Copyright Information){none=on}
      | Copyright info block.                                               
      |                                                                     
      | Place copyright information at the top of every subsystem in design.
      mask prompts: none "No parameters"
      mask help: Place copyright information at the top of every subsystem in design.
      mask Display:
      | NxtrConf = 'Nexteer Confidential';
      | 
      | sys = bdroot; %handle for the current model ("system")
      | first = get_param(sys,'Created');
      | first = first(end-3:end);  %year is last four digits
      | 
      | last = get_param(sys,'LastModifiedDate');
      | if isempty(last)
      |     last = datestr(now,'yyyy');
      | else
      |     last = last(end-3:end);
      | end
      | 
      | if strcmp(first,last)
      |     fprintf('%s -- Copyright %s Nexteer',NxtrConf,first)
      | else
      |     fprintf('%s -- %s%s- %s Nexteer',NxtrConf,char(169),first,last)
      | end
  Bit2Clr : Outport
  wires:
  Constant1/1 -> Bit2Clr/1

== system ES241A_MotAg2Meas/MotAg2Meas/MotAg2MeasPer1/AnalogMsbDiagnostics/TestFail/If Action Subsystem2 ==
  Action Port : ActionPort  ActionType=then
  Bit Set : simulink/Logic and Bit Operations/Bit Set  iBit=3
  Constant1 : Constant  Value=0  OutDataTypeStr=uint8
      settings: AttributesFormatString=%<OutDataTypeStr>
  CopyRight2 : Subsystem  Description=|  mask(Copyright Information){none=on}
      | Copyright info block.                                               
      |                                                                     
      | Place copyright information at the top of every subsystem in design.
      mask prompts: none "No parameters"
      mask help: Place copyright information at the top of every subsystem in design.
      mask Display:
      | NxtrConf = 'Nexteer Confidential';
      | 
      | sys = bdroot; %handle for the current model ("system")
      | first = get_param(sys,'Created');
      | first = first(end-3:end);  %year is last four digits
      | 
      | last = get_param(sys,'LastModifiedDate');
      | if isempty(last)
      |     last = datestr(now,'yyyy');
      | else
      |     last = last(end-3:end);
      | end
      | 
      | if strcmp(first,last)
      |     fprintf('%s -- Copyright %s Nexteer',NxtrConf,first)
      | else
      |     fprintf('%s -- %s%s- %s Nexteer',NxtrConf,char(169),first,last)
      | end
  Bit3Set : Outport
  wires:
  Bit Set/1 -> Bit3Set/1
  Constant1/1 -> Bit Set/1

== system ES241A_MotAg2Meas/MotAg2Meas/MotAg2MeasPer1/AnalogMsbDiagnostics/TestFail/If Action Subsystem3 ==
  Action Port : ActionPort  ActionType=else
  Constant1 : Constant  Value=0  OutDataTypeStr=uint8
      settings: AttributesFormatString=%<OutDataTypeStr>
  CopyRight2 : Subsystem  Description=|  mask(Copyright Information){none=on}
      | Copyright info block.                                               
      |                                                                     
      | Place copyright information at the top of every subsystem in design.
      mask prompts: none "No parameters"
      mask help: Place copyright information at the top of every subsystem in design.
      mask Display:
      | NxtrConf = 'Nexteer Confidential';
      | 
      | sys = bdroot; %handle for the current model ("system")
      | first = get_param(sys,'Created');
      | first = first(end-3:end);  %year is last four digits
      | 
      | last = get_param(sys,'LastModifiedDate');
      | if isempty(last)
      |     last = datestr(now,'yyyy');
      | else
      |     last = last(end-3:end);
      | end
      | 
      | if strcmp(first,last)
      |     fprintf('%s -- Copyright %s Nexteer',NxtrConf,first)
      | else
      |     fprintf('%s -- %s%s- %s Nexteer',NxtrConf,char(169),first,last)
      | end
  Bit3Clr : Outport
  wires:
  Constant1/1 -> Bit3Clr/1

== system ES241A_MotAg2Meas/MotAg2Meas/MotAg2MeasPer1/AnalogMsbDiagnostics/TestFail/Normal ==
  Action Port : ActionPort  ActionType=else
  Constant : Constant  Value=0  OutDataTypeStr=uint8
      settings: AttributesFormatString=%<OutDataTypeStr>
  CopyRight2 : Subsystem  Description=|  mask(Copyright Information){none=on}
      | Copyright info block.                                               
      |                                                                     
      | Place copyright information at the top of every subsystem in design.
      mask prompts: none "No parameters"
      mask help: Place copyright information at the top of every subsystem in design.
      mask Display:
      | NxtrConf = 'Nexteer Confidential';
      | 
      | sys = bdroot; %handle for the current model ("system")
      | first = get_param(sys,'Created');
      | if(isempty(first))
      |     first = datestr(now,'yyyy');
      | else
      |     first = first(end-3:end);  %year is last four digits
      | end
      | 
      | last = get_param(sys,'LastModifiedDate');
      | if isempty(last)
      |     last = datestr(now,'yyyy');
      | else
      |     last = last(end-3:end);
      | end
      | 
      | if strcmp(first,last)
      |     fprintf('%s -- Copyright %s Nexteer',NxtrConf,first)
      | else
      |     fprintf('%s -- %s%s- %s Nexteer',NxtrConf,char(169),first,last)
      | end
  Bit01Clr : Outport
  wires:
  Constant/1 -> Bit01Clr/1

== system ES241A_MotAg2Meas/MotAg2Meas/MotAg2MeasPer1/AnalogMsbDiagnostics/TestFail/SinCosMaxError ==
  Action Port : ActionPort  ActionType=elseif
  Bit Set : simulink/Logic and Bit Operations/Bit Set  iBit=1
  Constant : Constant  Value=0  OutDataTypeStr=uint8
  CopyRight2 : Subsystem  Description=|  mask(Copyright Information){none=on}
      | Copyright info block.                                               
      |                                                                     
      | Place copyright information at the top of every subsystem in design.
      mask prompts: none "No parameters"
      mask help: Place copyright information at the top of every subsystem in design.
      mask Display:
      | NxtrConf = 'Nexteer Confidential';
      | 
      | sys = bdroot; %handle for the current model ("system")
      | first = get_param(sys,'Created');
      | if(isempty(first))
      |     first = datestr(now,'yyyy');
      | else
      |     first = first(end-3:end);  %year is last four digits
      | end
      | 
      | last = get_param(sys,'LastModifiedDate');
      | if isempty(last)
      |     last = datestr(now,'yyyy');
      | else
      |     last = last(end-3:end);
      | end
      | 
      | if strcmp(first,last)
      |     fprintf('%s -- Copyright %s Nexteer',NxtrConf,first)
      | else
      |     fprintf('%s -- %s%s- %s Nexteer',NxtrConf,char(169),first,last)
      | end
  Bit1set : Outport
  wires:
  Bit Set/1 -> Bit1set/1
  Constant/1 -> Bit Set/1

== system ES241A_MotAg2Meas/MotAg2Meas/MotAg2MeasPer1/AnalogMsbDiagnostics/TestFail/SinCosMinError ==
  Action Port : ActionPort  ActionType=then
  Bit Set : simulink/Logic and Bit Operations/Bit Set  iBit=0
  Constant : Constant  Value=0  OutDataTypeStr=uint8
  CopyRight2 : Subsystem  Description=|  mask(Copyright Information){none=on}
      | Copyright info block.                                               
      |                                                                     
      | Place copyright information at the top of every subsystem in design.
      mask prompts: none "No parameters"
      mask help: Place copyright information at the top of every subsystem in design.
      mask Display:
      | NxtrConf = 'Nexteer Confidential';
      | 
      | sys = bdroot; %handle for the current model ("system")
      | first = get_param(sys,'Created');
      | if(isempty(first))
      |     first = datestr(now,'yyyy');
      | else
      |     first = first(end-3:end);  %year is last four digits
      | end
      | 
      | last = get_param(sys,'LastModifiedDate');
      | if isempty(last)
      |     last = datestr(now,'yyyy');
      | else
      |     last = last(end-3:end);
      | end
      | 
      | if strcmp(first,last)
      |     fprintf('%s -- Copyright %s Nexteer',NxtrConf,first)
      | else
      |     fprintf('%s -- %s%s- %s Nexteer',NxtrConf,char(169),first,last)
      | end
  Bit0Set : Outport
  wires:
  Constant/1 -> Bit Set/1
  Bit Set/1 -> Bit0Set/1

== system ES241A_MotAg2Meas/MotAg2Meas/MotAg2MeasPer1/AnalogMsbDiagnostics/TestPass/CopyRight2 ==

== system ES241A_MotAg2Meas/MotAg2Meas/MotAg2MeasPer1/MotAngleMechRevJdgmnt/TesOk_Fail/CopyRight2 ==

== system ES241A_MotAg2Meas/MotAg2Meas/MotAg2MeasPer1/MotAngleMechRevJdgmnt/TesOk_Pass/CopyRight2 ==

== system ES241A_MotAg2Meas/MotAg2Meas/MotAg2MeasPer1/MotPos_ArcTan/ATAN2/CopyRight2 ==

== system ES241A_MotAg2Meas/MotAg2Meas/MotAg2MeasPer1/MotPos_ArcTan/LimitMotAg2Meas/CopyRight2 ==

== system ES241A_MotAg2Meas/MotAg2Meas/MotAg2MeasPer1/MotPos_ArcTan/MotAg2MeclMeas/CopyRight2 ==

== system ES241A_MotAg2Meas/MotAg2Meas/MotAg2MeasPer1/MotPos_ArcTan/MotAg2MeclMeas/NegativePolarity ==
  MotAg2RawAg : Inport
  MotAg2OffsRevM : Inport  RequirementInfo={} %GIDa_c7a99eea_a52b_4795_9085_7616e57fb38f  Port=2
  Action Port : ActionPort  ActionType=else
  Add : Sum  Inputs=+-  OutDataTypeStr=Inherit: Inherit via back propagation
  Add1 : Sum  Inputs=+-
  Constant : Constant  OutDataTypeStr=single
  CopyRight2 : Subsystem  Description=|  mask(Copyright Information){none=on}
      | Copyright info block.                                               
      |                                                                     
      | Place copyright information at the top of every subsystem in design.
      mask prompts: none "No parameters"
      mask help: Place copyright information at the top of every subsystem in design.
      mask Display:
      | NxtrConf = 'Nexteer Confidential';
      | 
      | sys = bdroot; %handle for the current model ("system")
      | first = get_param(sys,'Created');
      | if(isempty(first))
      |     first = datestr(now,'yyyy');
      | else
      |     first = first(end-3:end);  %year is last four digits
      | end
      | 
      | last = get_param(sys,'LastModifiedDate');
      | if isempty(last)
      |     last = datestr(now,'yyyy');
      | else
      |     last = last(end-3:end);
      | end
      | 
      | if strcmp(first,last)
      |     fprintf('%s -- Copyright %s Nexteer',NxtrConf,first)
      | else
      |     fprintf('%s -- %s%s- %s Nexteer',NxtrConf,char(169),first,last)
      | end
  MotPosnMechRevM : Outport
  wires:
  Add/1 -> MotPosnMechRevM/1
  MotAg2RawAg/1 -> Add1/2
  Constant/1 -> Add1/1
  Add1/1 -> Add/1
  MotAg2OffsRevM/1 -> Add/2

== system ES241A_MotAg2Meas/MotAg2Meas/MotAg2MeasPer1/MotPos_ArcTan/MotAg2MeclMeas/PositivePolarity ==
  MotAg2RawAg : Inport
  MotAg2OffsRevM : Inport  RequirementInfo={} %GIDa_4ee2bc32_309e_4855_be7f_c9a84836da32  Port=2
  Action Port : ActionPort  ActionType=then
  Add : Sum  Inputs=+-  OutDataTypeStr=Inherit: Inherit via back propagation
  CopyRight2 : Subsystem  Description=|  mask(Copyright Information){none=on}
      | Copyright info block.                                               
      |                                                                     
      | Place copyright information at the top of every subsystem in design.
      mask prompts: none "No parameters"
      mask help: Place copyright information at the top of every subsystem in design.
      mask Display:
      | NxtrConf = 'Nexteer Confidential';
      | 
      | sys = bdroot; %handle for the current model ("system")
      | first = get_param(sys,'Created');
      | if(isempty(first))
      |     first = datestr(now,'yyyy');
      | else
      |     first = first(end-3:end);  %year is last four digits
      | end
      | 
      | last = get_param(sys,'LastModifiedDate');
      | if isempty(last)
      |     last = datestr(now,'yyyy');
      | else
      |     last = last(end-3:end);
      | end
      | 
      | if strcmp(first,last)
      |     fprintf('%s -- Copyright %s Nexteer',NxtrConf,first)
      | else
      |     fprintf('%s -- %s%s- %s Nexteer',NxtrConf,char(169),first,last)
      | end
  MotPosnMechRevM : Outport
  wires:
  Add/1 -> MotPosnMechRevM/1
  MotAg2RawAg/1 -> Add/1
  MotAg2OffsRevM/1 -> Add/2

== system ES241A_MotAg2Meas/MotAg2Meas/MotAg2MeasPer1/MotPos_ArcTan/QuadCorrect/CopyRight2 ==

== system ES241A_MotAg2Meas/MotAg2Meas/MotAg2MeasPer1/MotPos_ArcTan/SignalCorrect/CopyRight2 ==

== system ES241A_MotAg2Meas/MotAg2Meas/MotAg2MeasPer1/MotPos_ArcTan/SignalCorrect2/CopyRight2 ==
